simulink model "lab5"  (R2020b)
settings: Solver=VariableStepAuto  StartTime=0.0  StopTime=10.0  RelTol=1e-3
model workspace (MAT data in the model file):
  C = Simulink.Parameter
  C.Value = 10
  C.DataType = 'auto'
  C.Dimensions = [1 1]
  R = Simulink.Parameter
  R.Value = 10
  R.DataType = 'auto'
  R.Dimensions = [1 1]
settings Model: Creator=karth  LastModifiedBy=karth

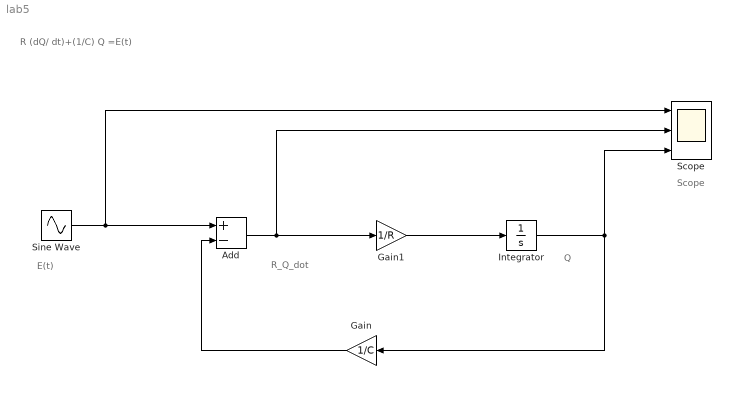
== system lab5 ==
  note: R (dQ/ dt)+(1/C) Q =E(t)
  note: Scope
  note: Q
  note: R_Q_dot
  note: E(t)
  Add : Sum  Inputs=+-
  Gain : Gain  Gain=1/C
  Gain1 : Gain  Gain=1/R
  Integrator : Integrator
  Scope : Scope  NumInputPorts=3
  Sine Wave : Sin  Amplitude=2*pi*100  SampleTime=0
  wires:
  Add/1 -> Scope/2, Gain1/1
  Gain1/1 -> Integrator/1
  Integrator/1 -> Gain/1, Scope/3
  Gain/1 -> Add/2
  Sine Wave/1 -> Scope/1, Add/1
